simulink library "wnnlib"  (R2021b)
settings: Solver=VariableStepAuto  StartTime=0.0  StopTime=10.0  RelTol=1e-3
PreLoadFcn:
  | DVG.Registry.addIconPackage(fullfile(matlabroot, 'toolbox', 'wnn', 'simulink', 'blockicons'))
undefined symbols (not defined in the file or in its folder): matdChol
libraries: simulink x5
settings Model: Creator=20214358  LastModifiedBy=20214358

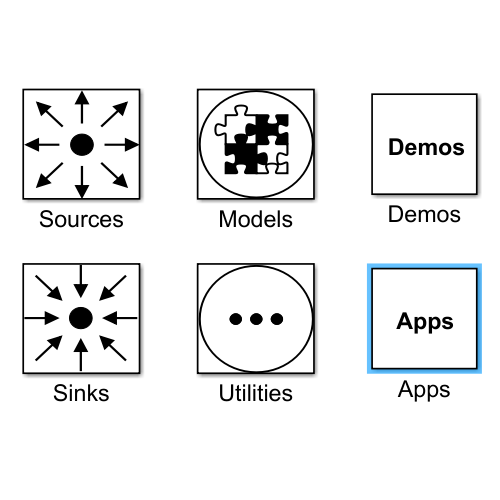
[thumbnail: Simulink's stored preview of the top-level diagram]
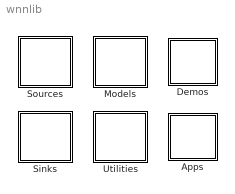
== system wnnlib ==
  Apps : Subsystem
      mask Display: disp('{\bf Apps}','interpreter','tex');
  Demos : Subsystem
      mask Display: disp('{\bf Demos}','interpreter','tex');
  Models : Subsystem
      mask Display: image('$imagefile'); % Use "Edit Image" on toolstrip to change.
  Sinks : Subsystem
      mask Display: image('$imagefile'); % Use "Edit Image" on toolstrip to change.
  Sources : Subsystem
      mask Display: image('$imagefile'); % Use "Edit Image" on toolstrip to change.
  Utilities : Subsystem
      mask Display: image('$imagefile'); % Use "Edit Image" on toolstrip to change.

== system wnnlib/Apps ==

== system wnnlib/Demos ==

== system wnnlib/Models ==
  VGRAM Array : Subsystem  mask(Virtual Generalized Random Access Memory (VGRAM)){array_id=0, min_mem_size=63, max_mem_size=64, min_dist=2, max_dist=8, pattern_length=16, output_dims=[16, 16], debug_flag=off}
      mask prompts: array_id "Array identifier"; min_mem_size "Minimum memory size"; max_mem_size "Maximum memory size"; min_dist "Minimum Hamming distance"; max_dist "Maximum Hamming distance"; pattern_length "Pattern length"; output_dims "Output dimensions"; debug_flag "Debug"
      mask init:
      | array_id=int32(array_id);
      | min_mem_size=int32(min_mem_size);
      | max_mem_size=int32(max_mem_size);
      | min_dist=int32(min_dist);
      | max_dist=int32(max_dist);
      | pattern_length=int32(pattern_length);
      | output_dims=int32(output_dims);
      | debug_flag=logical(debug_flag);
      mask Display:
      | disp('VGRAM Array')
      | port_label('input', 1, '{\bf b}','interpreter','tex')
      | port_label('input', 2, '{\bf b}^{\ast}','interpreter','tex')
      | port_label('input', 3, '\Delta{\bf h}^{\ast}','interpreter','tex')
      | port_label('input', 4, 'r/l','interpreter','tex')
      | port_label('output', 1,'{\bf h}','interpreter','tex')
      | port_label('trigger','\uparrow','interpreter','tex')

== system wnnlib/Sinks ==
  Scatter 2D : Subsystem  mask{axis_bounds=[0 1 0 1]}
      mask prompts: axis_bounds "Axis bounds"
      mask Display:
      | port_label('input', 1,'x','interpreter','tex')
      | port_label('input', 2,'y','interpreter','tex')
      | pos = get_param(gcb, 'Position');
      | width = pos(3) - pos(1);
      | height = pos(4) - pos(2);
      | x = [0.2 0.8 0.8 0.2 0.2]*width;
      | y = [0.2 0.2 0.8 0.8 0.2]*height;
      | plot(x,y)
      | x = [0 1 1 0 0]*width;
      | y = [0 0 1 1 0]*height;
      | plot(x,y)

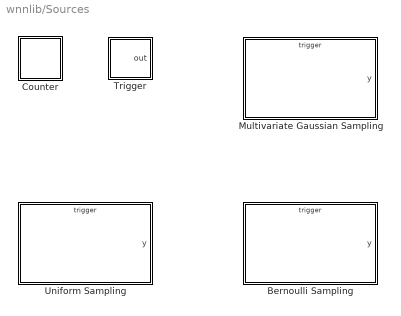
== system wnnlib/Sources ==
  Bernoulli Sampling : Subsystem  mask{nSamples=16, probability=0.5, nSeed=0}
      mask prompts: nSamples "Number of samples (n)"; probability "Probability of 1 outcome (p)"; nSeed "Seed"
      mask init:
      | nMins = zeros(1,nSamples);
      | nMaxs = ones(1,nSamples);
      | 
      | % Initialize seeds along dimensions
      | nSeeds = [1:nSamples] + nSeed;
      mask Display:
      | disp('{\bf y} \sim Be(n, p)','interpreter','tex');
      | port_label('output', 1,'{\bf y}','interpreter','tex')
      | port_label('trigger','\uparrow','interpreter','tex')
  Counter : Subsystem  mask{number_of_steps=10, sample_time=0}
      mask prompts: number_of_steps "Number of steps"; sample_time "Sample time"
      mask Display:
      | number_of_steps = get_param(gcb, 'number_of_steps');
      | patch([0 10 20 10], [10 20 10 0],[0.7294 0.8667 0.9490]);
      | disp('0{\rightarrow}'+string(number_of_steps),'interpreter','tex');
  Multivariate Gaussian Sampling : Subsystem  mask{vecdAvg=[1 1], matdCov=[2 1; 1 2], nSeed=0}
      mask prompts: vecdAvg "Average Vector"; matdCov "Covariance Matrix"; nSeed "Seed"
      mask init:
      | % Get number of dimensions
      | nDims=length(vecdAvg);
      | [nDims1, nDims2] = size(matdCov);
      | 
      | % Check number of dimensions
      | if nDims1 ~= nDims || nDims2 ~= nDims
      |     error('Covariance matrix and average vector dimensions are not compatible');
      | end
      | 
      | % Compute Cholesky decomposition of the covariance matrix
      | [matdChol,flag] = chol(matdCov);
      | 
      | % Check whether the covariance matrix is positive definite
      | if flag ~= 0
      |     error('Covariance matrix is not symmetric positive definite.');
      | end
      | 
      | % Initialize seeds along dimensions
      | nSeeds = [1:nDims] + nSeed;
      mask Display:
      | disp('{\bf y} \sim N({\bf \mu}, {\bf \Sigma})','interpreter','tex');
      | port_label('output', 1,'{\bf y}','interpreter','tex')
      | port_label('trigger','\uparrow','interpreter','tex')
  Trigger : Subsystem  mask{selected_steps=[0 0]}
      mask prompts: selected_steps "Selected steps"
      mask Display:
      | selected_steps = get_param(gcb, 'selected_steps');
      | patch([0 10 20 10], [10 20 10 0],[0.7294 0.8667 0.9490]);
      | 
      | selected_steps=strrep(selected_steps,'[','');
      | selected_steps=strrep(selected_steps,']','');
      | selected_steps=strrep(selected_steps,' ','|');
      | 
      | disp(selected_steps,'interpreter','tex');
      | port_label('output', 1,'\uparrow ','interpreter','tex');
  Uniform Sampling : Subsystem  mask{nSamples=16, min_value=0, max_value=10, nSeed=0}
      mask prompts: nSamples "Number of samples (n)"; min_value "Mininum value (a)"; max_value "Maximum value (b)"; nSeed "Seed"
      mask init:
      | % Check number of dimensions
      | if min_value >= max_value
      |     error('Invalid interval. Minimum value must be smaller than the maximum value.');
      | end
      | 
      | 
      | nMins = min_value*ones(1,nSamples);
      | nMaxs = max_value*ones(1,nSamples);
      | 
      | % Initialize seeds along dimensions
      | nSeeds = [1:nSamples] + nSeed;
      mask Display:
      | disp('{\bf y} \sim U(n, a, b)','interpreter','tex');
      | port_label('output', 1,'{\bf y}','interpreter','tex')
      | port_label('trigger','\uparrow','interpreter','tex')

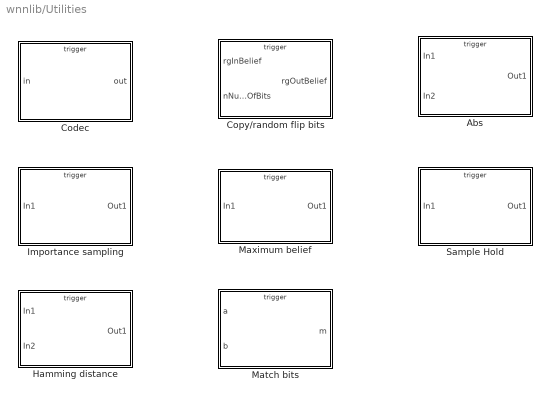
== system wnnlib/Utilities ==
  Abs : Subsystem
      mask Display:
      | disp('{\bf e} = \mid{\bf a} - {\bf b} \mid','interpreter','tex');
      | port_label('input', 1,'{\bf a}','interpreter','tex');
      | port_label('input', 2,'{\bf b}','interpreter','tex');
      | 
      | port_label('output', 1,'{\bf e}','interpreter','tex');
      | 
      | 
      | 
      | port_label('trigger','\uparrow','interpreter','tex');
  Codec : Subsystem  mask{codec_id=0, dense_vector_length=2, sparse_vector_length=2048, max_depth=16, learning_rate=0.001, min_splitting_volume=0.01, min_bounds=[0 0], max_bounds=[10 10], sparse_vectors_file=[], debug_flag=off, codec_type=Encoder, number_of_sparse_vectors=65536}
      mask prompts: codec_id "Codec id"; dense_vector_length "Dense vector length"; sparse_vector_length "Sparse vector length"; max_depth "Maximum kd-tree depth"; learning_rate "Learning rate"; min_splitting_volume "Minimum splitting volume"; min_bounds "Minimum bounds"; max_bounds "Maximum bounds"; sparse_vectors_file "Enter file name"; debug_flag "Debug"; codec_type "Codec type"; number_of_sparse_vectors "Number of sparse vectors"
      mask init:
      | codec_id=int32(codec_id);
      | dense_vector_length=int32(dense_vector_length);
      | sparse_vector_length=int32(sparse_vector_length);
      | max_depth=int32(max_depth);
      | learning_rate=double(learning_rate);
      | min_splitting_volume=double(min_splitting_volume);
      | min_bounds=double(min_bounds);
      | max_bounds=double(max_bounds);
      | sparse_vectors_file=char(sparse_vectors_file);
      | debug_flag=logical(debug_flag);
      | switch codec_type
      |     case 'Encoder'
      |         codec_type=int32(0);
      |     case 'Decoder'
      |         codec_type=int32(1);
      |     case 'OneHotEncoder'
      |         codec_type=int32(2);
      |     case 'OneHotDecoder'
      |         codec_type=int32(3);
      |     otherwise
      |         codec_type=[];
      | end
      | number_of_sparse_vectors=int32(number_of_sparse_vectors);
      mask TypeOptions codec_type: Encoder | Decoder | OneHotEncoder | OneHotDecoder
      mask Callback codec_type:
      | codec_type = get_param(gcb, 'codec_type');
      | 
      | switch codec_type
      |     case 'Encoder'
      |         set_param(gcb,'MaskVisibilities',{'on','on','on','on','on','on','on','on','on','on','on','off'});
      |     case 'Decoder'
      |         set_param(gcb,'MaskVisibilities',{'on','on','on','on','on','on','on','on','on','on','on','off'});
      |     case 'OneHotEncoder'
      |          set_param(gcb,'MaskVisibilities',{'on','on','on','on','on','on','on','on','on','on','on','on'});
      |     case 'OneHotDecoder'
      |          set_param(gcb,'MaskVisibilities',{'on','on','on','on','on','on','on','on','on','on','on','on'});
      |     otherwise
      |          set_param(gcb,'MaskVisibilities',{'on','on','on','on','on','on','on','on','on','on','on','off'});
      |  end
      mask DialogControl container Prompt: Sparse vectors file
      mask DialogControl browse_button Prompt: Browse file
      mask DialogControl browse_button Callback:
      | p = Simulink.Mask.get(gcb);
      | [fName, pName, ~] = uigetfile;
      | param = p.getParameter('sparse_vectors_file');
      | param.Value = char([pName, fName]);
      mask Display:
      | codec_type = get_param(gcb, 'codec_type');
      | 
      | switch codec_type
      |     case 'Encoder'
      |         disp('{\bf z} = {\bf m}_{y \rightarrow z}^{(' + string(get_param(gcb, 'codec_id'))+ ')}({\bf y})','interpreter','tex');
      |         port_label('input', 1,'{\bf y}','interpreter','tex');
      |         port_label('output', 1,'{\bf z}','interpreter','tex');
      |     case 'Decoder'
      |         disp('{\bf y} = {\bf m}_{z \rightarrow y}^{(' + string(get_param(gcb, 'codec_id'))+ ')}({\bf z})','interpreter','tex');
      |         port_label('input', 1,'{\bf z}','interpreter','tex');
      |         port_label('output', 1,'{\bf y}','interpreter','tex');
      |      case 'OneHotEncoder'
      |         disp('{\bf b} = {\bf m}_{z \rightarrow b}^{(' + string(get_param(gcb, 'codec_id'))+ ')}({\bf z})','interpreter','tex');
      |         port_label('input', 1,'{\bf z}','interpreter','tex');
      |         port_label('output', 1,'{\bf b}','interpreter','tex');
      |     case 'OneHotDecoder'
      |         disp('{\bf z} = {\bf m}_{b \rightarrow z}^{(' + string(get_param(gcb, 'codec_id'))+ ')}({\bf h})','interpreter','tex');
      |         port_label('input', 1,'{\bf b}','interpreter','tex');
      |         port_label('output', 1,'{\bf z}','interpreter','tex');
      |     otherwise
      |         disp('Invalid codec type','interpreter','tex');
      |         port_label('input', 1,'?','interpreter','tex');
      |         port_label('output', 1,'?','interpreter','tex');
      | end
      | 
      | port_label('trigger','\uparrow','interpreter','tex');
  Copy/random flip bits : Subsystem  TreatAsAtomicUnit=on
      mask help: Copy the the input belief to the output and flip the output values according to a given number of flips.
      mask Display:
      | disp('b^{\ast}_{i} \sim \{ b_{i}, \neg b_{i} \}','interpreter','tex');
      | port_label('input', 1,'{\bf b}','interpreter','tex')
      | port_label('input', 2,'n_{flips}','interpreter','tex')
      | port_label('output', 1,'{\bf b^{\ast}}','interpreter','tex')
      | port_label('trigger','\uparrow','interpreter','tex')
  Hamming distance : Subsystem
      mask Display:
      | disp('d_{h} = \Sigma_{i} a_{i} \oplus b_{i}','interpreter','tex');
      | port_label('input', 1,'{\bf a}','interpreter','tex')
      | port_label('input', 2,'{\bf b}','interpreter','tex')
      | port_label('output', 1,'d_{h}','interpreter','tex')
      | port_label('trigger','\uparrow','interpreter','tex')
  Importance sampling : Subsystem  TreatAsAtomicUnit=on  mask{nSamples=4}
      mask prompts: nSamples "Number of samples"
      mask help: Build an unnormalized belief from a histogram collecting the frequencies among a finite number of discrete states. The belief is encoded as a sparse binary sequence with the same length as the number of discrete states. However, it comprises a small number of ones (samples) among several zeros such that the likelihood of a discrete space being assigned to one is proportional to its corresponding frequency in the histogram.
      mask init:
      | assert(nSamples > 0, 'Number of samples must be greater than zero.')
      mask Display:
      | disp('b_{i} \sim \{ h_1,\ldots, h_n \}','interpreter','tex');
      | port_label('input', 1,'{\bf h}','interpreter','tex')
      | port_label('output', 1,'{\bf b}','interpreter','tex')
      | port_label('trigger','\uparrow','interpreter','tex')
  Match bits : Subsystem  TreatAsAtomicUnit=on  mask{nMatchTolerance=0}
      mask prompts: nMatchTolerance "Match tolerance"
      mask init:
      | nMatchTolerance=int32(nMatchTolerance);
      | assert(nMatchTolerance >=0, 'The match tolerance must be greater or equal zero');
      mask Display:
      | disp('\Sigma_{i} a_{i} \oplus b_{i} \leq tol','interpreter','tex');
      | port_label('input', 1,'{\bf a}','interpreter','tex')
      | port_label('input', 2,'{\bf b}','interpreter','tex')
      | port_label('output', 1,'y/n','interpreter','tex')
      | port_label('trigger','\uparrow','interpreter','tex')
  Maximum belief : Subsystem  TreatAsAtomicUnit=on
      mask Display:
      | disp('\ldots,0,1,0,\ldots','interpreter','tex');
      | port_label('input', 1,'{\bf h}','interpreter','tex')
      | port_label('output', 1,'{\bf b}','interpreter','tex')
      | port_label('trigger','\uparrow','interpreter','tex')
  Sample Hold : Subsystem  TreatAsAtomicUnit=on  mask{sample_time=0}
      mask prompts: sample_time "Sample time"
      mask Display:
      | disp('S/H','interpreter','tex');
      | 
      | port_label('trigger','\uparrow','interpreter','tex');

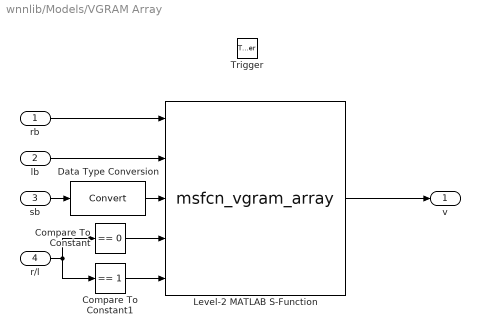
== system wnnlib/Models/VGRAM Array ==
  rb : Inport  LatchByDelayingOutsideSignal=on
  lb : Inport  Port=2  LatchByDelayingOutsideSignal=on
  sb : Inport  Port=3  LatchByDelayingOutsideSignal=on
  r/l : Inport  Port=4  LatchByDelayingOutsideSignal=on
  Trigger : TriggerPort  VariantControl=(inherit)  PortDimensions=1
  Compare To Constant : simulink/Logic and Bit Operations/Compare To Constant  relop===  const=0  OutDataTypeStr=boolean
  Compare To Constant1 : simulink/Logic and Bit Operations/Compare To Constant  relop===  const=1  OutDataTypeStr=boolean
  Data Type Conversion : DataTypeConversion
  Level-2 MATLAB S-Function : M-S-Function  FunctionName=msfcn_vgram_array  Parameters=array_id, output_dims, pattern_length, min_mem_size, max_mem_size, min_dist, max_dist, debug_flag
  v : Outport
  wires:
  rb/1 -> Level-2 MATLAB S-Function/1
  lb/1 -> Level-2 MATLAB S-Function/2
  Level-2 MATLAB S-Function/1 -> v/1
  Compare To Constant/1 -> Level-2 MATLAB S-Function/4
  Compare To Constant1/1 -> Level-2 MATLAB S-Function/5
  sb/1 -> Data Type Conversion/1
  r/l/1 -> Compare To Constant1/1, Compare To Constant/1
  Data Type Conversion/1 -> Level-2 MATLAB S-Function/3

== system wnnlib/Sinks/Scatter 2D ==
  x : Inport
  y : Inport  Port=2
  MATLAB Function : MATLAB Function  TreatAsAtomicUnit=on
  wires:
  y/1 -> MATLAB Function/2(y)
  x/1 -> MATLAB Function/1(x)

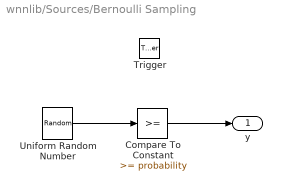
== system wnnlib/Sources/Bernoulli Sampling ==
  Trigger : TriggerPort  VariantControl=(inherit)  PortDimensions=1
  Compare To Constant : simulink/Logic and Bit Operations/Compare To Constant  relop=>=  const=probability  OutDataTypeStr=uint8
  Uniform Random Number : UniformRandomNumber  Minimum=nMins  Maximum=nMaxs  Seed=nSeeds
  y : Outport
  wires:
  Compare To Constant/1 -> y/1
  Uniform Random Number/1 -> Compare To Constant/1

== system wnnlib/Sources/Counter ==
  Counter : simulink/Sources/Counter Limited  uplimit=number_of_steps  tsamp=sample_time
  tag scope: current_step=global
  wires:
  Counter/1 -> [current_step]

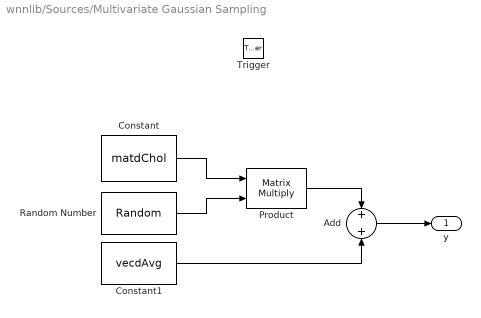
== system wnnlib/Sources/Multivariate Gaussian Sampling ==
  Trigger : TriggerPort  VariantControl=(inherit)  PortDimensions=1
  Add : Sum
  Constant : Constant  Value=matdChol  VectorParams1D=off
  Constant1 : Constant  Value=vecdAvg
  Product : Product  Multiplication=Matrix(*)
  Random Number : RandomNumber  Seed=nSeeds
  y : Outport
  wires:
  Add/1 -> y/1
  Constant1/1 -> Add/2
  Random Number/1 -> Product/2
  Product/1 -> Add/1
  Constant/1 -> Product/1

== system wnnlib/Sources/Trigger ==
  MATLAB Function : MATLAB Function  TreatAsAtomicUnit=on
  out : Outport
  wires:
  MATLAB Function/1(trigger) -> out/1
  [current_step] -> MATLAB Function/1(current_step)

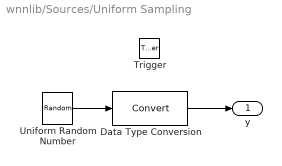
== system wnnlib/Sources/Uniform Sampling ==
  Trigger : TriggerPort  VariantControl=(inherit)  PortDimensions=1
  Data Type Conversion : DataTypeConversion  RndMeth=Round
  Uniform Random Number : UniformRandomNumber  Minimum=nMins  Maximum=nMaxs  Seed=nSeeds
  y : Outport
  wires:
  Data Type Conversion/1 -> y/1
  Uniform Random Number/1 -> Data Type Conversion/1

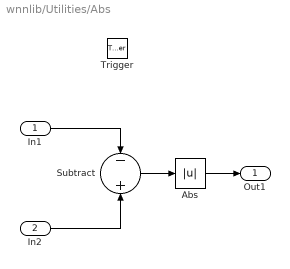
== system wnnlib/Utilities/Abs ==
  In1 : Inport
  In2 : Inport  Port=2
  Trigger : TriggerPort  VariantControl=(inherit)  PortDimensions=1
  Abs : Abs
  Subtract : Sum  Inputs=-+
  Out1 : Outport
  wires:
  Abs/1 -> Out1/1
  In2/1 -> Subtract/2
  Subtract/1 -> Abs/1
  In1/1 -> Subtract/1

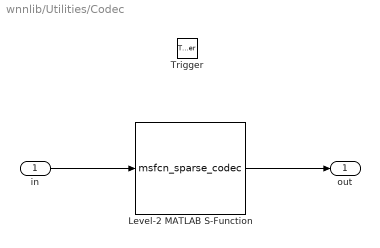
== system wnnlib/Utilities/Codec ==
  in : Inport
  Trigger : TriggerPort  VariantControl=(inherit)  PortDimensions=1
  Level-2 MATLAB S-Function : M-S-Function  FunctionName=msfcn_sparse_codec  Parameters=codec_id, dense_vector_length, sparse_vector_length, max_depth, learning_rate, min_splitting_volume, min_bounds, max_bounds, sparse_vectors_file, debug_flag, codec_type, number_of_sparse_vectors
  out : Outport
  wires:
  in/1 -> Level-2 MATLAB S-Function/1
  Level-2 MATLAB S-Function/1 -> out/1

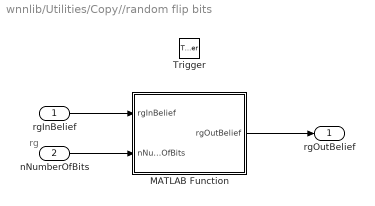
== system wnnlib/Utilities/Copy//random flip bits ==
  note: rg
  rgInBelief : Inport  OutDataTypeStr=uint8
  nNumberOfBits : Inport  Port=2  OutDataTypeStr=uint8
  Trigger : TriggerPort  VariantControl=(inherit)
  MATLAB Function : MATLAB Function  TreatAsAtomicUnit=on
  rgOutBelief : Outport  OutDataTypeStr=uint8
  wires:
  rgInBelief/1 -> MATLAB Function/1(rgInBelief)
  MATLAB Function/1(rgOutBelief) -> rgOutBelief/1
  nNumberOfBits/1 -> MATLAB Function/2(nNumberOfBits)

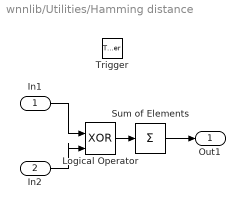
== system wnnlib/Utilities/Hamming distance ==
  In1 : Inport
  In2 : Inport  Port=2
  Trigger : TriggerPort  VariantControl=(inherit)  PortDimensions=1
  Logical Operator : Logic  Operator=XOR  IconShape=distinctive  AllPortsSameDT=off  OutDataTypeStr=boolean
  Sum of Elements : Sum  Inputs=+
  Out1 : Outport
  wires:
  In2/1 -> Logical Operator/2
  Logical Operator/1 -> Sum of Elements/1
  In1/1 -> Logical Operator/1
  Sum of Elements/1 -> Out1/1

== system wnnlib/Utilities/Importance sampling ==
  In1 : Inport
  Trigger : TriggerPort  VariantControl=(inherit)
  MATLAB Function : MATLAB Function  TreatAsAtomicUnit=on
  Out1 : Outport  OutDataTypeStr=uint8
  wires:
  In1/1 -> MATLAB Function/1(rgHistogram)
  MATLAB Function/1(rgBelief) -> Out1/1

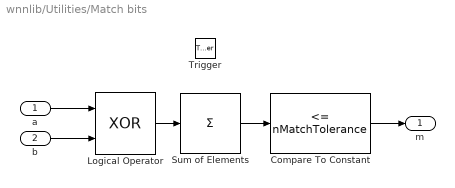
== system wnnlib/Utilities/Match bits ==
  a : Inport
  b : Inport  Port=2
  Trigger : TriggerPort  VariantControl=(inherit)
  Compare To Constant : simulink/Logic and Bit Operations/Compare To Constant  relop=<=  const=nMatchTolerance  OutDataTypeStr=boolean
  Logical Operator : Logic  Operator=XOR  AllPortsSameDT=off  OutDataTypeStr=boolean
  Sum of Elements : Sum  Inputs=+  AccumDataTypeStr=int32
  m : Outport
  wires:
  a/1 -> Logical Operator/1
  b/1 -> Logical Operator/2
  Logical Operator/1 -> Sum of Elements/1
  Compare To Constant/1 -> m/1
  Sum of Elements/1 -> Compare To Constant/1

== system wnnlib/Utilities/Maximum belief ==
  In1 : Inport
  Trigger : TriggerPort  VariantControl=(inherit)
  MATLAB Function : MATLAB Function  TreatAsAtomicUnit=on
  Out1 : Outport  OutDataTypeStr=uint8
  wires:
  MATLAB Function/1(rgBelief) -> Out1/1
  In1/1 -> MATLAB Function/1(rgHistogram)

== system wnnlib/Utilities/Sample Hold ==
  In1 : Inport
  Trigger : TriggerPort  VariantControl=(inherit)
  Zero-Order Hold : ZeroOrderHold  SampleTime=sample_time
  Out1 : Outport
  wires:
  In1/1 -> Zero-Order Hold/1
  Zero-Order Hold/1 -> Out1/1

== matlab function wnnlib/Utilities/Copy//random flip bits/MATLAB Function ==
  data: rgInBelief input; nNumberOfBits input; rgOutBelief output
function rgOutBelief = fcn(rgInBelief, nNumberOfBits)
% Copy the the input belief to the output and flip a given number of bits

% Get total number of discrete states
nDiscreteStates = numel(rgInBelief);

% Copy the input belief to the output
rgOutBelief = rgInBelief;

% Initialize the vector of selected indexes with zeros (invalid indexes)
rgSelectedIdxs = zeros(nNumberOfBits);
for i=1:nNumberOfBits
    % Select an index to flip
    while true
        nSelectedIdx = ceil(nDiscreteStates*rand);
        if isempty(find(rgSelectedIdxs==nSelectedIdx,1))
            break;
        end
    end
    % Store the selected index
    rgSelectedIdxs(i) = nSelectedIdx;

    % Flip the corresponding output value
    rgOutBelief(nSelectedIdx) = ~rgOutBelief(nSelectedIdx);
end

== matlab function wnnlib/Utilities/Importance sampling/MATLAB Function ==
  data: rgHistogram input; rgBelief output; nSamples parameter
function rgBelief = fcn(rgHistogram, nSamples)
% Build an unnormalized belief from a histogram collecting the frequencies
% among a finite number of discrete states. The belief is encoded as a 
% sparse binary sequence with the same length as the number of discrete
% states. However, it comprises a small number of ones (samples) among
% several zeros such that the likelihood of a discrete space being assigned
% to one is proportional to its corresponding frequency in the histogram.

% Get total number of discrete states
nDiscreteStates = numel(rgHistogram);

% Get the number of histogram dimensions
rgDims=size(rgHistogram);

% Initialize the unnormalized belief as all zeros
rgBelief = zeros(rgDims, 'uint8');

% Accumulate the histogram values
acc = sum(rgHistogram(:));

% Sanity check
if acc == 0
    idx = randi([1 nDiscreteStates], [1 nSamples]);
    rgBelief(idx) = uint8(1);
    return;
end

% Compute the normalization constant
k = 1/acc;

% Construct the probability mass function (p.m.f.)
rgPMF = k .* rgHistogram;

% Initialize the cummulative distribution function (c.d.f.)
rgCDF = zeros(rgDims);

% Construct the c.d.f.
rgCDF(1) = rgPMF(1);
for i=2:nDiscreteStates
    rgCDF(i) = rgCDF(i-1) + rgPMF(i);
end

% Draw a starting point
u1 = rand/nSamples;

% Start at the bottom of the c.d.f.
i = 1;

for j=1:nSamples
    % Set the threshold
    uj = u1 + (j-1)/nSamples;
    
    % Move along the c.d.f. to  
    while uj > rgCDF(i)
        i = i + 1;
    end

    % Assign a value one to the selected discrete state
    rgBelief(i) = uint8(1);
end

== matlab function wnnlib/Sources/Trigger/MATLAB Function ==
  data: current_step input; trigger output; selected_steps parameter
function trigger = fcn(current_step, selected_steps)

trigger = any(current_step==selected_steps);

== matlab function wnnlib/Utilities/Maximum belief/MATLAB Function ==
  data: rgHistogram input; rgBelief output
function rgBelief = fcn(rgHistogram)


% Get the number of histogram dimensions
rgDims=size(rgHistogram);

% Initialize the unnormalized belief as all zeros
rgBelief = zeros(rgDims, 'uint8');

% Get the index of the maximum value
[~, idx] = max(rgBelief);

% Assign a value one to the selected discrete state
rgBelief(idx) = uint8(1);

== matlab function wnnlib/Sinks/Scatter 2D/MATLAB Function ==
  data: x input; y input; axis_bounds parameter
function fcn(x,y,axis_bounds)

persistent hAxes

coder.extrinsic('scatter','axis'); 

if isempty(hAxes)
    figure();
    hAxes = gca;
    hold on
end

scatter(hAxes,x,y)
axis(axis_bounds);
axis equal;
